simulink model "chap5_3sim"  (Simulink 8.1)
settings: Solver=ode45  StartTime=0.0  StopTime=5  FixedStep=0.00000010  RelTol=1e-6
settings Model: Creator=ljk  LastModifiedBy=liujk  ExtModeTrigMode=oneshot  ExtModeArmWhenConnect=off
settings DataIOCC: LimitDataPoints=off  SignalLoggingName=sigsOut
settings OptimizationCC: BooleanDataType=off
settings DebuggingCC: SaveWithParameterizedLinksMsg=none  SignalResolutionControl=TryResolveAllWithWarning  SolverPrmCheckMsg=none  MultiTaskDSMMsg=warning  MultiTaskCondExecSysMsg=none  StrictBusMsg=None
settings HardwareCC: TargetUnknown=on
settings RTWCC: IncludeERTFirstTime=on

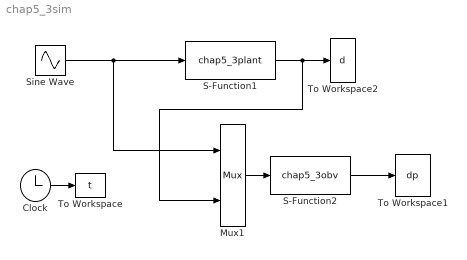
== system chap5_3sim ==
  Clock : Clock
  Mux1 : Mux  Inputs=2
  S-Function1 : S-Function  FunctionName=chap5_3plant  EnableBusSupport=off
  S-Function2 : S-Function  FunctionName=chap5_3obv  EnableBusSupport=off
  Sine Wave : Sin  SampleTime=0
  To Workspace : ToWorkspace  VariableName=t  SampleTime=-1
  To Workspace1 : ToWorkspace  VariableName=dp  SampleTime=-1
  To Workspace2 : ToWorkspace  VariableName=d  SampleTime=-1
  wires:
  Clock/1 -> To Workspace/1
  Mux1/1 -> S-Function2/1
  S-Function2/1 -> To Workspace1/1
  Sine Wave/1 -> S-Function1/1, Mux1/1
  S-Function1/1 -> Mux1/2, To Workspace2/1
